simulink library "dspparest3"  (Simulink 8.0)
settings: Solver=ode45  SolverMode=SingleTasking  StartTime=0.0  StopTime=10.0  RelTol=1e-3
values from neighbouring files (symbols this model uses):
  A = localGetVal(inData.InstanceData, 'A', '[1 1 0 0]')    [dspddes3Transform.m]    (also in msepred.m = eye(L) - 2*mu*Lam + mu^2*(Lam^2*(kurt+2)+dLam*dLam'))
  D = D + B    [rebuffer_delay.m]
libraries: dspmtrx3 x20, dspsigattribs x11, dspsolvers x3, dspstat3 x1
settings Model: RequirementInfo=9  FPTRunName=Active  Creator=don  LastModifiedBy=lij  CovMetricSettings=d  ExtModeAutoUpdateStatusClock=off

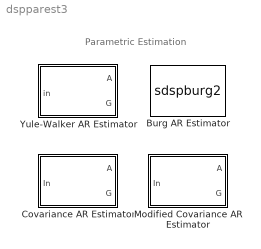
== system dspparest3 ==
  note: Parametric Estimation
  Burg AR Estimator : S-Function  FunctionName=sdspburg2  Parameters=fcn, inheritOrder, ord  EnableBusSupport=off  mask(Burg AR Estimator){fcn=A, inheritOrder=on, ord=4}
      mask prompts: fcn "Output(s):"; inheritOrder "Inherit estimation order from input dimensions"; ord "Estimation order:"
      mask help: Frame-based parametric AR estimation using the Burg maximum entropy method. Outputs AR model coefficients A and/or reflection coefficients K, plus the model gain, G.
      mask init:
      | s = dspblkburg2('icon');
      mask Help: eval('blocksethelp');
      mask StyleString: popup(A and K|A|K),checkbox,edit
      mask CallbackString: |dspblkburg2|
      mask Display:
      | disp('Burg AR\nEstimator');
      | port_label('output',s.o1,s.o1s);
      | port_label('output',s.o2,s.o2s);
      | port_label('output',s.o3,s.o3s);
  Covariance AR Estimator : Subsystem  mask(Covariance AR Estimator){P=4}
      mask prompts: P "Estimation order:"
      mask help: Frame-based parametric AR estimation using the Covariance method. The AR model coefficients are given in A and the gain is given in G.
      mask init:
      | if ~isreal(P) || (P <= 0) || (P~=floor(P))
      |    err.eID = 'dsp:dspparest3:InvalidEstimationOrder';
      |    err.msg = ['The ''Estimation order'' parameter must be a real positive integer.'];
      |    error(err.eID,err.msg);
      | end
      mask Help: eval('blocksethelp');
      mask Display: disp('Cov AR\nEstimator')
  Modified Covariance AR Estimator : Subsystem  mask(Modified Covariance AR Estimator){P=4}
      mask prompts: P "Estimation order:"
      mask help: Frame-based parametric AR estimation using the Modified Covariance method. The AR model coefficients are given in A and the gain is given in G.
      mask init: same as dspparest3/Covariance AR Estimator
      mask Help: eval('blocksethelp');
      mask Display: disp('MCov AR\nEstimator')
  Yule-Walker AR Estimator : Subsystem  mask(Yule-Walker AR Estimator){ywArOutType=A, inheritOrder=on, ord=4}
      mask prompts: ywArOutType "Output(s):"; inheritOrder "Inherit estimation order from input dimensions"; ord "Estimation order:"
      mask help: Frame-based parametric AR estimation using the Yule-Walker method. The AR model coefficients are given in A (polynomial coefficients) and/or K (reflection coefficients). The square of the model gain is given in G.
      mask init:
      | acf = dspblkywestim('computeVars',ord);
      | dspblkywestim('init');
      mask Help: eval('blocksethelp');
      mask StyleString: popup(A and K|A|K),checkbox,edit
      mask CallbackString: |dspblkywestim|
      mask Display: disp('Yule AR\nEstimator')

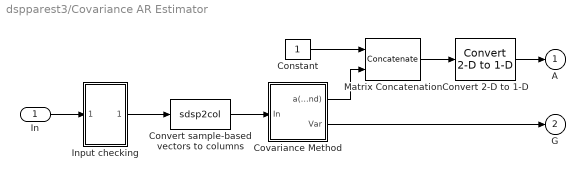
== system dspparest3/Covariance AR Estimator ==
  In : Inport
  Constant : Constant  OutDataTypeStr=Inherit: Inherit via back propagation
  Convert 2-D to 1-D : dspsigattribs/Convert 2-D to 1-D
  Convert sample-based vectors to columns : S-Function  FunctionName=sdsp2col  EnableBusSupport=off
  Covariance Method : Subsystem
  Input checking : Subsystem
  Matrix Concatenation : Concatenate  Mode=Multidimensional array
  A : Outport  InitialOutput=0
  G : Outport  Port=2  InitialOutput=0
  wires:
  Matrix Concatenation/1 -> Convert 2-D to 1-D/1
  Covariance Method/1(a(2:end)) -> Matrix Concatenation/2
  Constant/1 -> Matrix Concatenation/1
  Covariance Method/2(Var) -> G/1
  In/1 -> Input checking/1(In1)
  Convert sample-based vectors to columns/1 -> Covariance Method/1(In)
  Convert 2-D to 1-D/1 -> A/1
  Input checking/1(Out1) -> Convert sample-based vectors to columns/1

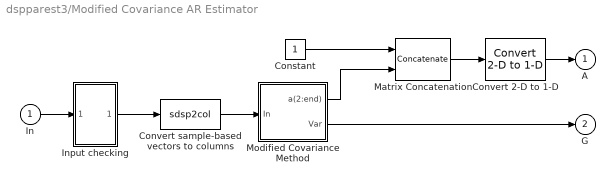
== system dspparest3/Modified Covariance AR Estimator ==
  In : Inport
  Constant : Constant  OutDataTypeStr=Inherit: Inherit via back propagation
  Convert 2-D to 1-D : dspsigattribs/Convert 2-D to 1-D
  Convert sample-based vectors to columns : S-Function  FunctionName=sdsp2col  EnableBusSupport=off
  Input checking : Subsystem
  Matrix Concatenation : Concatenate  Mode=Multidimensional array
  Modified Covariance Method : Subsystem
  A : Outport  InitialOutput=0
  G : Outport  Port=2  InitialOutput=0
  wires:
  Modified Covariance Method/2(Var) -> G/1
  Constant/1 -> Matrix Concatenation/1
  Matrix Concatenation/1 -> Convert 2-D to 1-D/1
  Modified Covariance Method/1(a(2:end)) -> Matrix Concatenation/2
  In/1 -> Input checking/1(In1)
  Convert sample-based vectors to columns/1 -> Modified Covariance Method/1(In)
  Convert 2-D to 1-D/1 -> A/1
  Input checking/1(Out1) -> Convert sample-based vectors to columns/1

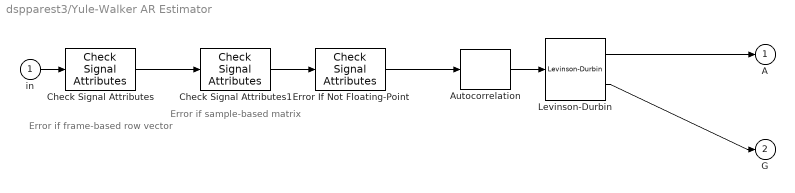
== system dspparest3/Yule-Walker AR Estimator ==
  note: Error if
      | sample-based
      | matrix
  note: Error if
      | frame-based
      | row vector
  in : Inport
  Autocorrelation : dspstat3/Autocorrelation  AllPositiveLags=on  maxlag=acf  bias=Biased  domain=Time  outputDataTypeStr=Inherit: Same as accumulator  outputLastDataTypeStr=Inherit: Same as accumulator  outputMin=[]  outputMax=[]  accumDataTypeStr=Inherit: Same as product output  accumLastDataTypeStr=Inherit: Same as product output  roundingMode=Floor  overflowMode=off
  Check Signal Attributes : dspsigattribs/Check Signal Attributes  SystemSampleTime=-1  SigAttribCheckMethod=Matches attributes exactly  Complexity=Ignore  Frame=Frame-based  DimsCheckMethod=Is...  Dimensions=Row vector (2-D)  DatatypeCheckMethod=Ignore  DatatypeGeneral=Boolean  DtypeFloatSpecific=Any floating-point  DtypeFixedSpecific=Any fixed-point  DtypeIntSpecific=Any integer  SampleMode=Ignore
  Check Signal Attributes1 : dspsigattribs/Check Signal Attributes  SystemSampleTime=-1  SigAttribCheckMethod=Matches attributes exactly  Complexity=Ignore  Frame=Sample-based  DimsCheckMethod=Is...  Dimensions=Full matrix (2-D)  DatatypeCheckMethod=Ignore  DatatypeGeneral=Boolean  DtypeFloatSpecific=Any floating-point  DtypeFixedSpecific=Any fixed-point  DtypeIntSpecific=Any integer  SampleMode=Ignore
  Error If Not Floating-Point : dspsigattribs/Check Signal Attributes  SystemSampleTime=-1  SigAttribCheckMethod=Does not match attributes exactly  Complexity=Ignore  Frame=Ignore  DimsCheckMethod=Ignore  Dimensions=1-D  DatatypeCheckMethod=Is...  DatatypeGeneral=Floating-point  DtypeFloatSpecific=Any floating-point  DtypeFixedSpecific=Any fixed-point  DtypeIntSpecific=Any integer  SampleMode=Ignore
  Levinson-Durbin : dspsolvers/Levinson-Durbin  coeffOutFcn=OBSOLETE  coeffOutFcnActive=A  outP=on  zeroInpHandling=on  firstCoeffMode=Binary point scaling  firstCoeffWordLength=16  firstCoeffFracLength=15  firstCoeffDataTypeStr=fixdt(1,16,15)  firstCoeffLastDataTypeStr=fixdt(1,16,15)  firstCoeffMin=[]  firstCoeffMax=[]  secondCoeffMode=Binary point scaling  secondCoeffWordLength=16  secondCoeffFracLength=15  secondCoeffDataTypeStr=fixdt(1,16,15)  secondCoeffLastDataTypeStr=fixdt(1,16,15)  secondCoeffMin=[]  secondCoeffMax=[]  outputMin=[]  outputMax=[]  accumMode=User-defined  accumWordLength=32  accumFracLength=30  accumDataTypeStr=fixdt(1,32,30)  accumLastDataTypeStr=fixdt(1,32,30)  prodOutputMode=User-defined  prodOutputWordLength=32  prodOutputFracLength=30  prodOutputDataTypeStr=fixdt(1,32,30)  prodOutputLastDataTypeStr=fixdt(1,32,30)  roundingMode=Floor  overflowMode=off
      settings: allowOverrides=off
  A : Outport  InitialOutput=0
  G : Outport  Port=2
  wires:
  Levinson-Durbin/2 -> G/1
  Autocorrelation/1 -> Levinson-Durbin/1
  Levinson-Durbin/1 -> A/1
  in/1 -> Check Signal Attributes/1
  Check Signal Attributes1/1 -> Error If Not Floating-Point/1
  Error If Not Floating-Point/1 -> Autocorrelation/1
  Check Signal Attributes/1 -> Check Signal Attributes1/1

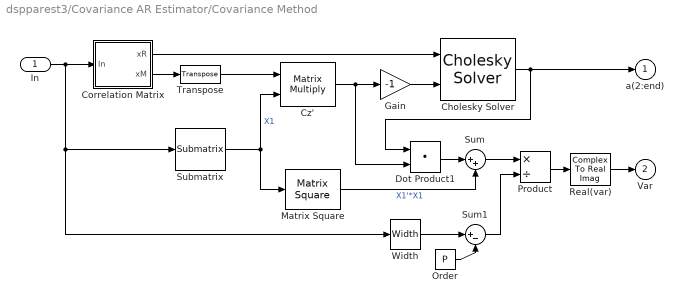
== system dspparest3/Covariance AR Estimator/Covariance Method ==
  In : Inport
  Cholesky Solver : dspsolvers/Cholesky Solver  errmode=Warning
  Correlation Matrix : Subsystem
  Cz' : Product  Multiplication=Matrix(*)
  Dot Product1 : DotProduct  OutDataTypeStr=Inherit: Inherit via internal rule
  Gain : Gain  Gain=-1  SaturateOnIntegerOverflow=on  OutDataTypeStr=Inherit: Same as input  ParamDataTypeStr=Inherit: Same as input
  Matrix Square : dspmtrx3/Matrix Square  OutMin=[]  OutMax=[]
  Order : Constant  Value=P  OutDataTypeStr=Inherit: Inherit via back propagation
  Product : Product  Inputs=*/  SaturateOnIntegerOverflow=on  InputSameDT=on  OutDataTypeStr=Inherit: Same as first input
  Real(var) : ComplexToRealImag  Output=Real
  Submatrix : dspmtrx3/Submatrix  RowSpan=Range of rows  RowStartMode=Index  RowStartIndex=P+1  RowEndMode=Last  RowEndIndex=1  ColSpan=All columns  ColStartMode=First  ColStartIndex=1  ColEndMode=Last  ColEndIndex=1
  Sum : Sum  Inputs=|++  SaturateOnIntegerOverflow=on  InputSameDT=on  OutDataTypeStr=Inherit: Same as first input
  Sum1 : Sum  Inputs=|+-  SaturateOnIntegerOverflow=on  InputSameDT=on  OutDataTypeStr=Inherit: Same as first input
  Transpose : dspmtrx3/Transpose  Hermitian=on  overflowFlag=on
  Width : Width  OutDataTypeMode=All ports same datatype
  a(2:end) : Outport  InitialOutput=0
  Var : Outport  Port=2  InitialOutput=0
  wires:
  Order/1 -> Sum1/2
  Width/1 -> Sum1/1
  In/1 -> Correlation Matrix/1(In), Submatrix/1, Width/1
  Cz'/1 -> Dot Product1/2, Gain/1
  Submatrix/1 -> Cz'/2, Matrix Square/1  "X1"
  Correlation Matrix/2(xM) -> Transpose/1
  Transpose/1 -> Cz'/1
  Gain/1 -> Cholesky Solver/2
  Correlation Matrix/1(xR) -> Cholesky Solver/1
  Cholesky Solver/1 -> Dot Product1/1, a(2:end)/1
  Dot Product1/1 -> Sum/1
  Matrix Square/1 -> Sum/2  "X1'*X1"
  Sum/1 -> Product/1
  Product/1 -> Real(var)/1
  Real(var)/1 -> Var/1
  Sum1/1 -> Product/2

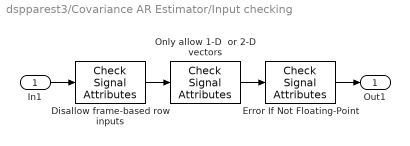
== system dspparest3/Covariance AR Estimator/Input checking ==
  In1 : Inport
  Disallow frame-based row inputs : dspsigattribs/Check Signal Attributes  SigAttribCheckMethod=Matches attributes exactly  Complexity=Ignore  Frame=Frame-based  DimsCheckMethod=Is...  Dimensions=Row vector (2-D)  DatatypeCheckMethod=Ignore  DatatypeGeneral=Boolean  DtypeFloatSpecific=Any floating-point  DtypeFixedSpecific=Any fixed-point  DtypeIntSpecific=Any integer  SampleMode=Ignore
  Error If Not Floating-Point : dspsigattribs/Check Signal Attributes  SigAttribCheckMethod=Does not match attributes exactly  Complexity=Ignore  Frame=Ignore  DimsCheckMethod=Ignore  Dimensions=1-D  DatatypeCheckMethod=Is...  DatatypeGeneral=Floating-point  DtypeFloatSpecific=Any floating-point  DtypeFixedSpecific=Any fixed-point  DtypeIntSpecific=Any integer  SampleMode=Ignore
  Only allow 1-D  or 2-D vectors : dspsigattribs/Check Signal Attributes  SigAttribCheckMethod=Does not match attributes exactly  Complexity=Ignore  Frame=Ignore  DimsCheckMethod=Is...  Dimensions=Vector (1-D or 2-D)  DatatypeCheckMethod=Ignore  DatatypeGeneral=Boolean  DtypeFloatSpecific=Any floating-point  DtypeFixedSpecific=Any fixed-point  DtypeIntSpecific=Any integer  SampleMode=Ignore
  Out1 : Outport
  wires:
  Disallow frame-based row inputs/1 -> Only allow 1-D  or 2-D vectors/1
  Only allow 1-D  or 2-D vectors/1 -> Error If Not Floating-Point/1
  In1/1 -> Disallow frame-based row inputs/1
  Error If Not Floating-Point/1 -> Out1/1

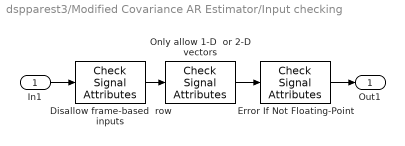
== system dspparest3/Modified Covariance AR Estimator/Input checking ==
  In1 : Inport
  Disallow frame-based  row inputs : dspsigattribs/Check Signal Attributes  SigAttribCheckMethod=Matches attributes exactly  Complexity=Ignore  Frame=Frame-based  DimsCheckMethod=Is...  Dimensions=Row vector (2-D)  DatatypeCheckMethod=Ignore  DatatypeGeneral=Boolean  DtypeFloatSpecific=Any floating-point  DtypeFixedSpecific=Any fixed-point  DtypeIntSpecific=Any integer  SampleMode=Ignore
  Error If Not Floating-Point : dspsigattribs/Check Signal Attributes  SigAttribCheckMethod=Does not match attributes exactly  Complexity=Ignore  Frame=Ignore  DimsCheckMethod=Ignore  Dimensions=1-D  DatatypeCheckMethod=Is...  DatatypeGeneral=Floating-point  DtypeFloatSpecific=Any floating-point  DtypeFixedSpecific=Any fixed-point  DtypeIntSpecific=Any integer  SampleMode=Ignore
  Only allow 1-D  or 2-D vectors : dspsigattribs/Check Signal Attributes  SigAttribCheckMethod=Does not match attributes exactly  Complexity=Ignore  Frame=Ignore  DimsCheckMethod=Is...  Dimensions=Vector (1-D or 2-D)  DatatypeCheckMethod=Ignore  DatatypeGeneral=Boolean  DtypeFloatSpecific=Any floating-point  DtypeFixedSpecific=Any fixed-point  DtypeIntSpecific=Any integer  SampleMode=Ignore
  Out1 : Outport
  wires:
  Only allow 1-D  or 2-D vectors/1 -> Error If Not Floating-Point/1
  Disallow frame-based  row inputs/1 -> Only allow 1-D  or 2-D vectors/1
  In1/1 -> Disallow frame-based  row inputs/1
  Error If Not Floating-Point/1 -> Out1/1

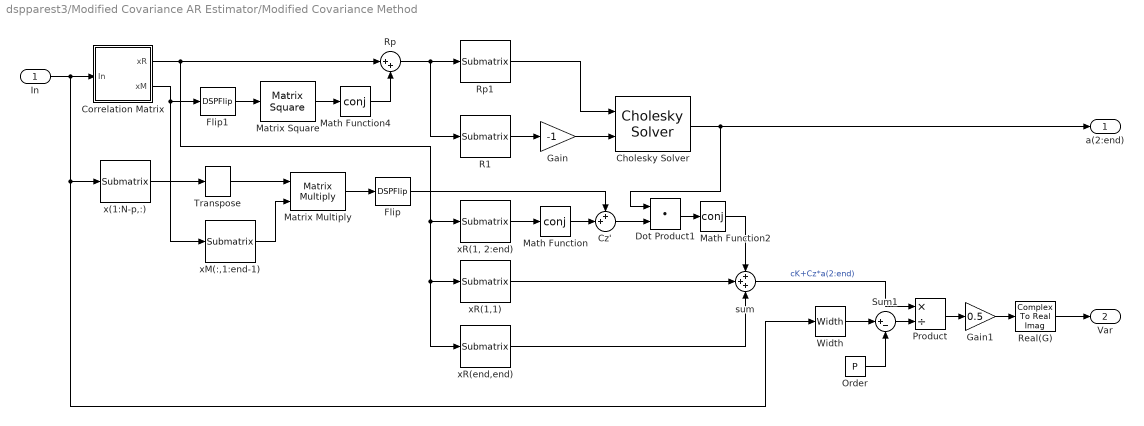
== system dspparest3/Modified Covariance AR Estimator/Modified Covariance Method ==
  In : Inport
  Cholesky Solver : dspsolvers/Cholesky Solver  errmode=Warning
  Correlation Matrix : Subsystem
  Cz' : Sum  Inputs=++|  SaturateOnIntegerOverflow=on  InputSameDT=on  OutDataTypeStr=Inherit: Same as first input
  Dot Product1 : DotProduct  OutDataTypeStr=Inherit: Inherit via internal rule
  Flip : DSPFlip  dim=Rows
  Flip1 : DSPFlip  dim=Rows
  Gain : Gain  Gain=-1  SaturateOnIntegerOverflow=on  OutDataTypeStr=Inherit: Same as input  ParamDataTypeStr=Inherit: Same as input
  Gain1 : Gain  Gain=0.5  SaturateOnIntegerOverflow=on  OutDataTypeStr=Inherit: Same as input  ParamDataTypeStr=Inherit: Same as input
  Math Function : Math  Operator=conj  SaturateOnIntegerOverflow=on
  Math Function2 : Math  Operator=conj  SaturateOnIntegerOverflow=on
  Math Function4 : Math  Operator=conj  SaturateOnIntegerOverflow=on
  Matrix Square : dspmtrx3/Matrix Square  OutMin=[]  OutMax=[]
  Matrix Multiply : Product  Multiplication=Matrix(*)
  Order : Constant  Value=P  OutDataTypeStr=Inherit: Inherit via back propagation
  Product : Product  Inputs=*/  SaturateOnIntegerOverflow=on  InputSameDT=on  OutDataTypeStr=Inherit: Same as first input
  R1 : dspmtrx3/Submatrix  RowSpan=Range of rows  RowStartMode=Index  RowStartIndex=2  RowEndMode=Last  RowEndIndex=P  ColSpan=One column  ColStartMode=First  ColStartIndex=2  ColEndMode=Last  ColEndIndex=1
  Real(G) : ComplexToRealImag  Output=Real
  Rp : Sum  Inputs=|++  SaturateOnIntegerOverflow=on  InputSameDT=on  OutDataTypeStr=Inherit: Same as first input
  Rp1 : dspmtrx3/Submatrix  RowSpan=Range of rows  RowStartMode=Index  RowStartIndex=2  RowEndMode=Last  RowEndIndex=P  ColSpan=Range of columns  ColStartMode=Index  ColStartIndex=2  ColEndMode=Last  ColEndIndex=1
  Sum1 : Sum  Inputs=|+-  SaturateOnIntegerOverflow=on  InputSameDT=on  OutDataTypeStr=Inherit: Same as first input
  Transpose : dspmtrx3/Transpose  Hermitian=on  overflowFlag=on
  Width : Width  OutDataTypeMode=All ports same datatype
  sum : Sum  Inputs=+++  SaturateOnIntegerOverflow=on  InputSameDT=on  OutDataTypeStr=Inherit: Same as first input
  x(1:N-p,:) : dspmtrx3/Submatrix  RowSpan=Range of rows  RowStartMode=First  RowStartIndex=1  RowEndMode=Offset from last  RowEndIndex=P  ColSpan=All columns  ColStartMode=First  ColStartIndex=1  ColEndMode=Index  ColEndIndex=P
  xM(:,1:end-1) : dspmtrx3/Submatrix  RowSpan=All rows  RowStartMode=First  RowStartIndex=1  RowEndMode=Offset from last  RowEndIndex=P  ColSpan=Range of columns  ColStartMode=First  ColStartIndex=1  ColEndMode=Offset from last  ColEndIndex=1
  "xR(1, 2:end)" : dspmtrx3/Submatrix  RowSpan=One row  RowStartMode=First  RowStartIndex=2  RowEndMode=Last  RowEndIndex=P  ColSpan=Range of columns  ColStartMode=Index  ColStartIndex=2  ColEndMode=Last  ColEndIndex=1
  xR(1,1) : dspmtrx3/Submatrix  RowSpan=One row  RowStartMode=First  RowStartIndex=2  RowEndMode=Index  RowEndIndex=1  ColSpan=One column  ColStartMode=First  ColStartIndex=2  ColEndMode=Last  ColEndIndex=1
  xR(end,end) : dspmtrx3/Submatrix  RowSpan=One row  RowStartMode=Last  RowStartIndex=0  RowEndMode=Last  RowEndIndex=1  ColSpan=One column  ColStartMode=Last  ColStartIndex=0  ColEndMode=Last  ColEndIndex=1
  a(2:end) : Outport
  Var : Outport  Port=2
  wires:
  sum/1 -> Product/1  "cK+Cz*a(2:end)"
  Product/1 -> Gain1/1
  Order/1 -> Sum1/2
  Width/1 -> Sum1/1
  Sum1/1 -> Product/2
  Correlation Matrix/1(xR) -> "xR(1, 2:end)"/1, xR(1,1)/1, xR(end,end)/1, Rp/1
  In/1 -> Correlation Matrix/1(In), Width/1, x(1:N-p,:)/1
  Math Function4/1 -> Rp/2
  Flip1/1 -> Matrix Square/1
  xM(:,1:end-1)/1 -> Matrix Multiply/2
  Math Function/1 -> Cz'/2
  "xR(1, 2:end)"/1 -> Math Function/1
  Flip/1 -> Cz'/1
  Matrix Multiply/1 -> Flip/1
  Dot Product1/1 -> Math Function2/1
  Cz'/1 -> Dot Product1/2
  Matrix Square/1 -> Math Function4/1
  Correlation Matrix/2(xM) -> xM(:,1:end-1)/1, Flip1/1
  Transpose/1 -> Matrix Multiply/1
  x(1:N-p,:)/1 -> Transpose/1
  Rp/1 -> Rp1/1, R1/1
  Cholesky Solver/1 -> a(2:end)/1, Dot Product1/1
  R1/1 -> Gain/1
  Gain/1 -> Cholesky Solver/2
  xR(1,1)/1 -> sum/2
  xR(end,end)/1 -> sum/3
  Math Function2/1 -> sum/1
  Gain1/1 -> Real(G)/1
  Real(G)/1 -> Var/1
  Rp1/1 -> Cholesky Solver/1

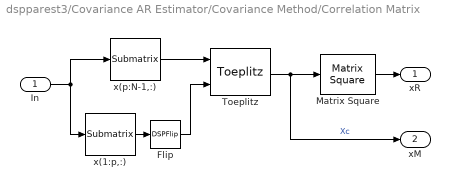
== system dspparest3/Covariance AR Estimator/Covariance Method/Correlation Matrix ==
  In : Inport
  Flip : DSPFlip
  Matrix Square : dspmtrx3/Matrix Square  OutMin=[]  OutMax=[]
  Toeplitz : dspmtrx3/Toeplitz  Symmetric=off  overflowFlag=on
  x(1:p,:) : dspmtrx3/Submatrix  RowSpan=Range of rows  RowStartMode=First  RowStartIndex=P  RowEndMode=Index  RowEndIndex=P  ColSpan=All columns  ColStartMode=First  ColStartIndex=1  ColEndMode=Last  ColEndIndex=1
  x(p:N-1,:) : dspmtrx3/Submatrix  RowSpan=Range of rows  RowStartMode=Index  RowStartIndex=P  RowEndMode=Offset from last  RowEndIndex=1  ColSpan=All columns  ColStartMode=First  ColStartIndex=1  ColEndMode=Last  ColEndIndex=1
  xR : Outport
  xM : Outport  Port=2
  wires:
  x(1:p,:)/1 -> Flip/1
  x(p:N-1,:)/1 -> Toeplitz/1
  Toeplitz/1 -> Matrix Square/1, xM/1  "Xc"
  In/1 -> x(p:N-1,:)/1, x(1:p,:)/1
  Matrix Square/1 -> xR/1
  Flip/1 -> Toeplitz/2

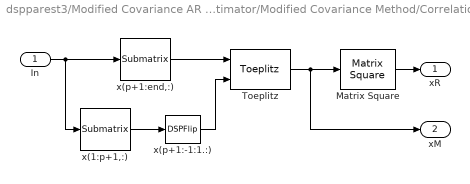
== system dspparest3/Modified Covariance AR Estimator/Modified Covariance Method/Correlation Matrix ==
  In : Inport
  Matrix Square : dspmtrx3/Matrix Square  OutMin=[]  OutMax=[]
  Toeplitz : dspmtrx3/Toeplitz  Symmetric=off  overflowFlag=on
  x(1:p+1,:) : dspmtrx3/Submatrix  RowSpan=Range of rows  RowStartMode=First  RowStartIndex=P  RowEndMode=Index  RowEndIndex=P+1  ColSpan=All columns  ColStartMode=First  ColStartIndex=1  ColEndMode=Last  ColEndIndex=1
  x(p+1:-1:1.:) : DSPFlip
  x(p+1:end,:) : dspmtrx3/Submatrix  RowSpan=Range of rows  RowStartMode=Index  RowStartIndex=P+1  RowEndMode=Last  RowEndIndex=1  ColSpan=All columns  ColStartMode=First  ColStartIndex=1  ColEndMode=Last  ColEndIndex=1
  xR : Outport
  xM : Outport  Port=2
  wires:
  x(1:p+1,:)/1 -> x(p+1:-1:1.:)/1
  x(p+1:-1:1.:)/1 -> Toeplitz/2
  Toeplitz/1 -> xM/1, Matrix Square/1
  In/1 -> x(1:p+1,:)/1, x(p+1:end,:)/1
  Matrix Square/1 -> xR/1
  x(p+1:end,:)/1 -> Toeplitz/1
